simulink model "altitude_control"  (R2017a)
settings: Solver=VariableStepAuto  StartTime=0.0  StopTime=20  RelTol=1e-3
values from neighbouring files (symbols this model uses):
  a_theta1 = -P.rho*Va^2*P.c*P.S_wing/(2*P.Jy)*P.C_m_q*P.c/(2*Va)    [compute_gains.m]
  a_theta2 = -P.rho*Va^2*P.c*P.S_wing*P.C_m_alpha/(2*P.Jy)    [compute_gains.m]
  a_theta3 = P.rho*Va^2*P.c*P.S_wing/(2*P.Jy)*P.C_m_delta_e    [compute_gains.m]
  delta_e_max = 45*pi/180    (= 0.785398163397)    [compute_gains.m]
  Va = sqrt(x_trim(4)^2+x_trim(5)^2+x_trim(6))    [compute_gains.m]    (also in forces_moments.m = P.Va0; forces_moments_v2.m = P.Va0)
undefined symbols (not defined in the file or in its folder): P
settings Model: Creator=pizzaslayer  LastModifiedBy=pizzaslayer

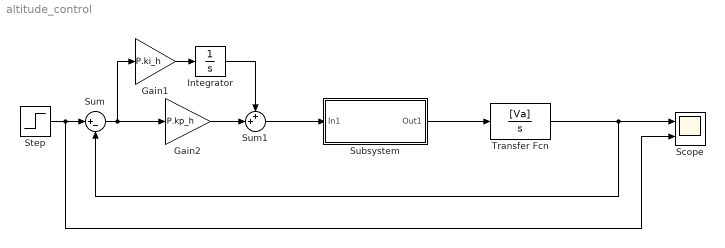
== system altitude_control ==
  Gain1 : Gain  Gain=P.ki_h
  Gain2 : Gain  Gain=P.kp_h
  Integrator : Integrator
  Scope : Scope  NumInputPorts=2
  Step : Step  Time=0  After=10  SampleTime=0
  Subsystem : Subsystem
  Sum : Sum  Inputs=|+-
  Sum1 : Sum  Inputs=++|
  Transfer Fcn : TransferFcn  Numerator=[Va]  Denominator=[1 0]
  wires:
  Step/1 -> Scope/2, Sum/1
  Sum/1 -> Gain1/1, Gain2/1
  Gain1/1 -> Integrator/1
  Integrator/1 -> Sum1/1
  Gain2/1 -> Sum1/2
  Transfer Fcn/1 -> Sum/2, Scope/1
  Subsystem/1(Out1) -> Transfer Fcn/1
  Sum1/1 -> Subsystem/1(In1)

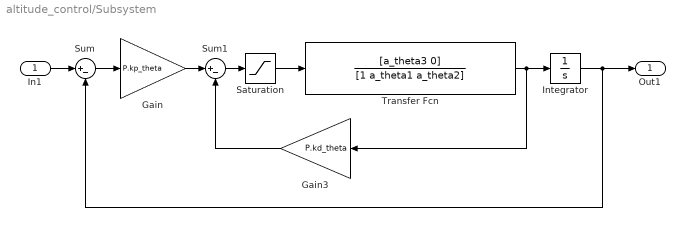
== system altitude_control/Subsystem ==
  In1 : Inport
  Gain : Gain  Gain=P.kp_theta
  Gain3 : Gain  Gain=P.kd_theta
  Integrator : Integrator
  Saturation : Saturate  UpperLimit=delta_e_max  LowerLimit=-delta_e_max
  Sum : Sum  Inputs=|+-
  Sum1 : Sum  Inputs=|+-
  Transfer Fcn : TransferFcn  Numerator=[a_theta3 0]  Denominator=[1 a_theta1 a_theta2]
  Out1 : Outport
  wires:
  Sum1/1 -> Saturation/1
  Integrator/1 -> Out1/1, Sum/2
  Transfer Fcn/1 -> Integrator/1, Gain3/1
  Gain/1 -> Sum1/1
  Saturation/1 -> Transfer Fcn/1
  Sum/1 -> Gain/1
  Gain3/1 -> Sum1/2
  In1/1 -> Sum/1
